simulink model "AM"  (R2020b)
settings: Solver=VariableStepAuto  StartTime=0.0  StopTime=10.0  RelTol=1e-3
settings Model: Creator=Lenovo  LastModifiedBy=Lenovo

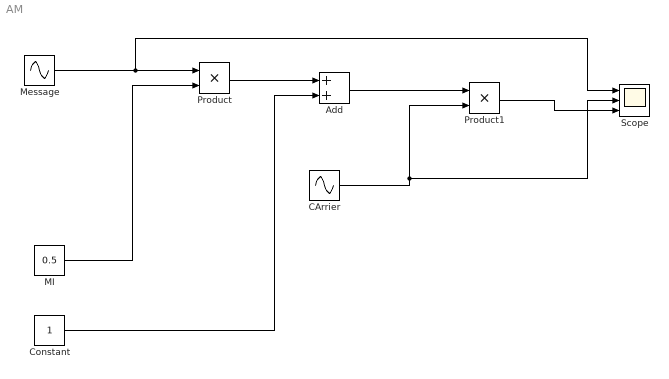
== system AM ==
  Add : Sum
  CArrier : Sin  Frequency=2*pi*25  SampleTime=0
  Constant : Constant
  MI : Constant  Value=0.5
  Message : Sin  Frequency=2*pi*5  SampleTime=0
  Product : Product
  Product1 : Product
  Scope : Scope  NumInputPorts=3
  wires:
  Message/1 -> Scope/1, Product/1
  MI/1 -> Product/2
  Product/1 -> Add/1
  Constant/1 -> Add/2
  Add/1 -> Product1/1
  CArrier/1 -> Scope/2, Product1/2
  Product1/1 -> Scope/3
